simulink model "ThresholdCalibration6CH_UI"  (R2018b)
settings: Solver=VariableStepAuto  StartTime=0.0  StopTime=inf  RelTol=1e-3
libraries: simulink x16, dspstat3 x8, aerolibanimutils x1, dspnetwork x1
settings Model: Creator=Bruger  LastModifiedBy=Jonathan E. Schmidt

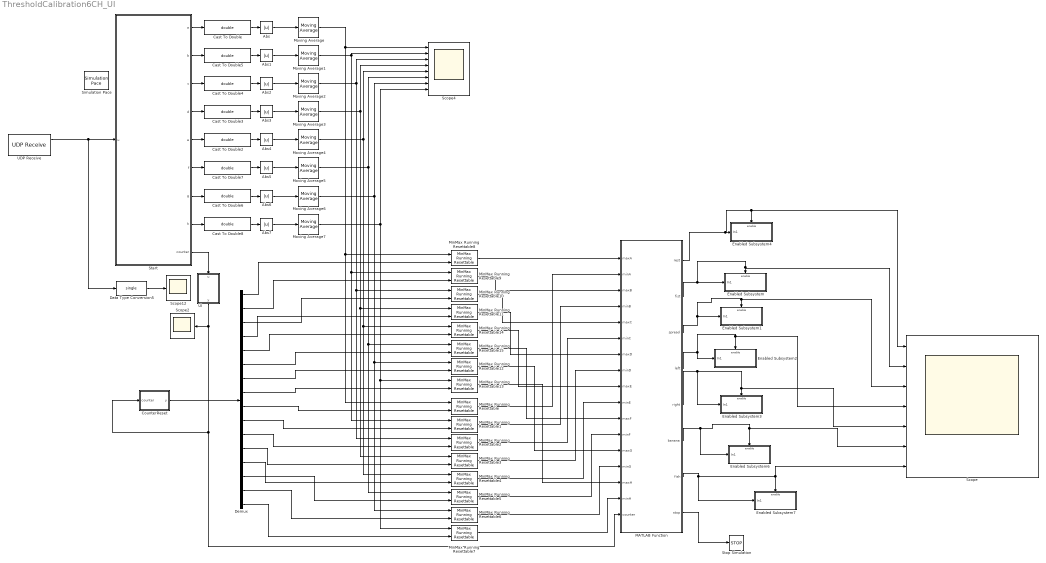
== system ThresholdCalibration6CH_UI ==
  Abs{,1..7} (8 alike) : Abs
  Cast To Double{,2..8} (8 alike) : DataTypeConversion  OutDataTypeStr=double
  "CounterReset " : MATLAB Function  TreatAsAtomicUnit=on
  Data Type Conversion5 : DataTypeConversion  OutDataTypeStr=single
  Demux : Demux  Outputs=16
  Enabled Subsystem : Subsystem  TreatAsAtomicUnit=on
  Enabled Subsystem1 : Subsystem  TreatAsAtomicUnit=on
  Enabled Subsystem2 : Subsystem  TreatAsAtomicUnit=on
  Enabled Subsystem3 : Subsystem  TreatAsAtomicUnit=on
  Enabled Subsystem4 : Subsystem  TreatAsAtomicUnit=on
  Enabled Subsystem6 : Subsystem  TreatAsAtomicUnit=on
  Enabled Subsystem7 : Subsystem  TreatAsAtomicUnit=on
  MATLAB Function : MATLAB Function  TreatAsAtomicUnit=on
  MinMax Running Resettable{,1..7} (8 alike) : simulink/Math Operations/MinMax Running Resettable  Function=min  vinit=1000
  MinMax Running Resettable{8..15} (8 alike) : simulink/Math Operations/MinMax Running Resettable  Function=max  vinit=0
  Moving Average{,1..7} (8 alike) : dspstat3/Moving Average  Method=Sliding window  ForgettingFactorPort=off  SpecifyWindowLength=on  WindowLength=50  ForgettingFactor=0.9  SimulateUsing=Code generation
  Scope : Scope  NumInputPorts=7
  Scope12 : Scope
  Scope2 : Scope
  Scope4 : Scope  NumInputPorts=8
  Simulation Pace : aerolibanimutils/Simulation Pace  SimulationPace=1  SleepMode=Auto  OutputPaceError=off  SampleTime=1/30
  "Start " : MATLAB Function  TreatAsAtomicUnit=on
  Stop Simulation : Stop
  UDP Receive : dspnetwork/UDP Receive  localURL='0.0.0.0'  localPort=54000  remoteURL='0.0.0.0'  remotePort=-1  recvBufferSize=128  dims=255  signalDatatype=int8  isVarSize=off  showBlockingTime=off  blockingTime=0  sampletime=0.02  blockPlatform=[]
      settings: SourceProductName=DSP System Toolbox  SourceProductBaseCode=DS
  UI : MATLAB Function  TreatAsAtomicUnit=on
  wires:
  UDP Receive/1 -> Data Type Conversion5/1, "Start "/1(u)
  Data Type Conversion5/1 -> Scope12/1
  Cast To Double/1 -> Abs/1
  "Start "/1(a) -> Cast To Double/1
  "Start "/2(b) -> Cast To Double5/1
  Cast To Double5/1 -> Abs1/1
  "Start "/3(c) -> Cast To Double4/1
  Cast To Double4/1 -> Abs2/1
  "Start "/4(d) -> Cast To Double3/1
  Cast To Double3/1 -> Abs3/1
  "Start "/5(e) -> Cast To Double2/1
  Cast To Double2/1 -> Abs4/1
  "Start "/6(f) -> Cast To Double7/1
  Cast To Double7/1 -> Abs5/1
  "Start "/7(g) -> Cast To Double6/1
  Cast To Double6/1 -> Abs6/1
  "Start "/8(h) -> Cast To Double8/1
  Cast To Double8/1 -> Abs7/1
  Moving Average1/1 -> MinMax Running Resettable9/1, MinMax Running Resettable1/1, Scope4/2
  Moving Average2/1 -> MinMax Running Resettable10/1, MinMax Running Resettable2/1, Scope4/3
  Moving Average3/1 -> MinMax Running Resettable11/1, MinMax Running Resettable3/1, Scope4/4
  Moving Average4/1 -> MinMax Running Resettable14/1, MinMax Running Resettable4/1, Scope4/5
  Moving Average5/1 -> MinMax Running Resettable15/1, MinMax Running Resettable5/1, Scope4/6
  Moving Average6/1 -> MinMax Running Resettable12/1, MinMax Running Resettable6/1, Scope4/7
  Moving Average7/1 -> MinMax Running Resettable7/1, MinMax Running Resettable13/1, Scope4/8
  Abs/1 -> Moving Average/1
  Abs1/1 -> Moving Average1/1
  Abs2/1 -> Moving Average2/1
  Abs3/1 -> Moving Average3/1
  Abs4/1 -> Moving Average4/1
  Abs5/1 -> Moving Average5/1
  Abs6/1 -> Moving Average6/1
  Abs7/1 -> Moving Average7/1
  MinMax Running Resettable8/1 -> MATLAB Function/1(maxA)
  MinMax Running Resettable/1 -> MATLAB Function/2(minA)
  MinMax Running Resettable9/1 -> MATLAB Function/3(maxB)
  MinMax Running Resettable1/1 -> MATLAB Function/4(minB)
  MinMax Running Resettable10/1 -> MATLAB Function/5(maxC)
  MinMax Running Resettable2/1 -> MATLAB Function/6(minC)
  MinMax Running Resettable11/1 -> MATLAB Function/7(maxD)
  MinMax Running Resettable3/1 -> MATLAB Function/8(minD)
  MinMax Running Resettable14/1 -> MATLAB Function/9(maxE)
  MinMax Running Resettable4/1 -> MATLAB Function/10(minE)
  MinMax Running Resettable15/1 -> MATLAB Function/11(maxF)
  MinMax Running Resettable5/1 -> MATLAB Function/12(minF)
  MinMax Running Resettable12/1 -> MATLAB Function/13(maxG)
  MinMax Running Resettable6/1 -> MATLAB Function/14(minG)
  MinMax Running Resettable13/1 -> MATLAB Function/15(maxH)
  MinMax Running Resettable7/1 -> MATLAB Function/16(minH)
  Demux/1 -> MinMax Running Resettable8/2
  Demux/2 -> MinMax Running Resettable9/2
  Demux/3 -> MinMax Running Resettable10/2
  Demux/4 -> MinMax Running Resettable11/2
  Demux/5 -> MinMax Running Resettable14/2
  Demux/6 -> MinMax Running Resettable15/2
  Demux/7 -> MinMax Running Resettable12/2
  Demux/8 -> MinMax Running Resettable13/2
  Demux/9 -> MinMax Running Resettable/2
  Demux/10 -> MinMax Running Resettable1/2
  Demux/11 -> MinMax Running Resettable2/2
  Demux/12 -> MinMax Running Resettable3/2
  Demux/13 -> MinMax Running Resettable4/2
  Demux/14 -> MinMax Running Resettable5/2
  Demux/15 -> MinMax Running Resettable6/2
  Demux/16 -> MinMax Running Resettable7/2
  Moving Average/1 -> MinMax Running Resettable/1, MinMax Running Resettable8/1, Scope4/1
  "CounterReset "/1(y) -> Demux/1
  MATLAB Function/2(fist) -> Scope/2, Enabled Subsystem/Enable, Enabled Subsystem/1(In1)
  MATLAB Function/3(spread) -> Scope/3, Enabled Subsystem1/Enable, Enabled Subsystem1/1(In1)
  MATLAB Function/4(left) -> Scope/4, Enabled Subsystem2/Enable, Enabled Subsystem2/1(In1)
  MATLAB Function/5(right) -> Enabled Subsystem3/1(In1), Scope/5, Enabled Subsystem3/Enable
  MATLAB Function/6(banana) -> Scope/6, Enabled Subsystem6/Enable, Enabled Subsystem6/1(In1)
  MATLAB Function/7(fish) -> Scope/7, Enabled Subsystem7/Enable, Enabled Subsystem7/1(In1)
  MATLAB Function/8(stop) -> Stop Simulation/1
  MATLAB Function/1(rest) -> Scope/1, Enabled Subsystem4/Enable, Enabled Subsystem4/1(In1)
  "Start "/9(counter) -> UI/1(u)
  UI/1(y) -> "CounterReset "/1(counter), MATLAB Function/17(counter), Scope2/1

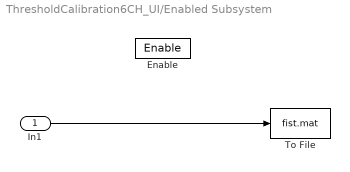
== system ThresholdCalibration6CH_UI/Enabled Subsystem ==
  In1 : Inport
  Enable : EnablePort
  To File : ToFile  Filename=fist.mat  MatrixName=fist
  wires:
  In1/1 -> To File/1

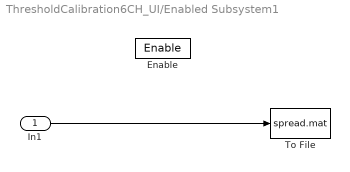
== system ThresholdCalibration6CH_UI/Enabled Subsystem1 ==
  In1 : Inport
  Enable : EnablePort
  To File : ToFile  Filename=spread.mat  MatrixName=spread
  wires:
  In1/1 -> To File/1

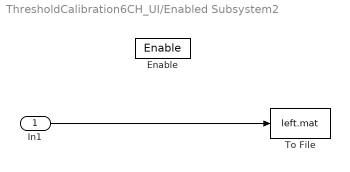
== system ThresholdCalibration6CH_UI/Enabled Subsystem2 ==
  In1 : Inport
  Enable : EnablePort
  To File : ToFile  Filename=left.mat  MatrixName=left
  wires:
  In1/1 -> To File/1

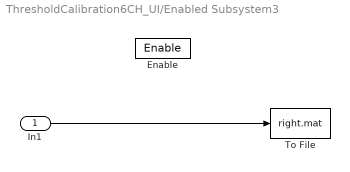
== system ThresholdCalibration6CH_UI/Enabled Subsystem3 ==
  In1 : Inport
  Enable : EnablePort
  To File : ToFile  Filename=right.mat  MatrixName=minMax
  wires:
  In1/1 -> To File/1

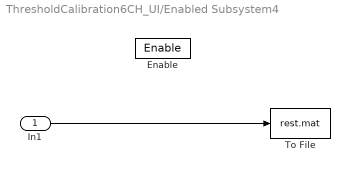
== system ThresholdCalibration6CH_UI/Enabled Subsystem4 ==
  In1 : Inport
  Enable : EnablePort
  To File : ToFile  Filename=rest.mat  MatrixName=fist
  wires:
  In1/1 -> To File/1

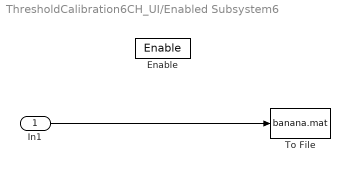
== system ThresholdCalibration6CH_UI/Enabled Subsystem6 ==
  In1 : Inport
  Enable : EnablePort
  To File : ToFile  Filename=banana.mat  MatrixName=fish
  wires:
  In1/1 -> To File/1

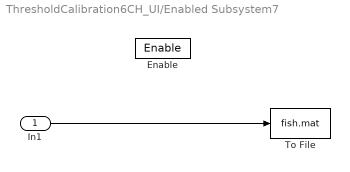
== system ThresholdCalibration6CH_UI/Enabled Subsystem7 ==
  In1 : Inport
  Enable : EnablePort
  To File : ToFile  Filename=fish.mat  MatrixName=fish
  wires:
  In1/1 -> To File/1

== matlab function ThresholdCalibration6CH_UI/UI ==
  data: u input; y output
function y = fcn(u)
coder.extrinsic('uipanel')
coder.extrinsic('uicontrol')

% persistent h1 h2 h4 counter;

persistent h1 h2 h4;


% if isempty(counter)
%     counter=0;
% else
%     counter=counter+1;
% end

if isempty(h1)
    close all;
    h1 = figure(...
    'PaperUnits','inches',...
    'Units','characters',...
    'Position',[100 20 130.4 26.8461538461538],...
    'PaperSize',[8.5 11],...
    'PaperType','usletter');

    h2 = uipanel(...
    'Parent',h1,...
    'Units','characters',...
    'Title','Current task',...
    'Position',[9.8 17.6153846153846 41.4 5.30769230769231],...
    'FontSize',10);

    h4 = uipanel(...
    'Parent',h1,...
    'Units','characters',...
    'Title','Upcoming task',...
    'Position',[9.8 9.92307692307692 41.4 5.30769230769231],...
    'FontSize',10);

    h6 = uipanel(...
    'Parent',h1,...
    'Units','characters',...
    'Title','Instructions',...
    'Position',[55.2 2.23076923076923 67.6 20.6923076923077],...
    'FontSize',10);

    h7 = uicontrol(...
    'Parent',h6,...
    'Units','characters',...
    'HorizontalAlignment','left',...
    'String',{  'The calibration process has 6 steps. Each step takes 5 seconds that are followed by 4 seconds of a rest time. The calibration starts with 10 seconds of rest. The user is expected to already be resting his/her arm once the program starts.'; blanks(0); 'The user is expected to perform the gestures in the following order:'; '1. Relaxed'; '2. Spread'; '3. Wave left'; '4. Wave right'; '5. Fist pull-back '; '6. Fist ' },...
    'Style','text',...
    'Position',[4.4 1.38461538461538 55 17.5384615384615],...
    'FontSize',9);
end

% % % % % % % % % % % % % % % % % % % % % % % % % % % % % % % % % % % % % % % % % % % % % % % % % %
% % % % % % % % % % % % % % % % % % % % % % % % % % % % % % % % % % % % % % % % % % % % % % % % % % 
% % % % % % % % % % % % % % % % % % % % % % % % % % % % % % % % % % % % % % % % % % % % % % % % % % 
% % % % % % % % % % % % % % % % % % % % % % % % % % % % % % % % % % % % % % % % % % % % % % % % % % 

switch u
    case 1
        h3 = uicontrol(...
        'Parent',h2,...
        'Units','characters',...
        'String',{  'Relaxed' },...
        'Style','text',...
        'FontSize',10,...
        'Position',[3 1.30769230769231 35 2]);
    
        h5 = uicontrol(...
        'Parent',h4,...
        'Units','characters',...
        'String',{  'Rest' },...
        'Style','text',...
        'FontSize',10,...
        'Position',[2.2 1.38461538461538 35 2]);
    
    case 250
        h3 = uicontrol(...
        'Parent',h2,...
        'Units','characters',...
        'String',{  'Rest' },...
        'Style','text',...
        'FontSize',10,...
        'Position',[3 1.30769230769231 35 2]);
    
        h5 = uicontrol(...
        'Parent',h4,...
        'Units','characters',...
        'String',{  'Spread' },...
        'Style','text',...
        'FontSize',10,...
        'Position',[2.2 1.38461538461538 35 2]);
    
    case 450
        h3 = uicontrol(...
        'Parent',h2,...
        'Units','characters',...
        'String',{  'Spread' },...
        'Style','text',...
        'FontSize',10,...
        'Position',[3 1.30769230769231 35 2]);
    
        h5 = uicontrol(...
        'Parent',h4,...
        'Units','characters',...
        'String',{  'Rest' },...
        'Style','text',...
        'FontSize',10,...
        'Position',[2.2 1.38461538461538 35 2]);
    
    case 750 
        h3 = uicontrol(...
        'Parent',h2,...
        'Units','characters',...
        'String',{  'Rest' },...
        'Style','text',...
        'FontSize',10,...
        'Position',[3 1.30769230769231 35 2]);
    
        h5 = uicontrol(...
        'Parent',h4,...
        'Units','characters',...
        'String',{  'Wave left' },...
        'Style','text',...
        'FontSize',10,...
        'Position',[2.2 1.38461538461538 35 2]);

    case 950
        h3 = uicontrol(...
        'Parent',h2,...
        'Units','characters',...
        'String',{  'Wave left' },...
        'Style','text',...
        'FontSize',10,...
        'Position',[3 1.30769230769231 35 2]);
    
        h5 = uicontrol(...
        'Parent',h4,...
        'Units','characters',...
        'String',{  'Rest' },...
        'Style','text',...
        'FontSize',10,...
        'Position',[2.2 1.38461538461538 35 2]);

    case 1250
        h3 = uicontrol(...
        'Parent',h2,...
        'Units','characters',...
        'String',{  'Rest' },...
        'Style','text',...
        'FontSize',10,...
        'Position',[3 1.30769230769231 35 2]);
    
        h5 = uicontrol(...
        'Parent',h4,...
        'Units','characters',...
        'String',{  'Wave right' },...
        'Style','text',...
        'FontSize',10,...
        'Position',[2.2 1.38461538461538 35 2]);
    
    case 1450
        h3 = uicontrol(...
        'Parent',h2,...
        'Units','characters',...
        'String',{  'Wave right' },...
        'Style','text',...
        'FontSize',10,...
        'Position',[3 1.30769230769231 35 2]);
    
        h5 = uicontrol(...
        'Parent',h4,...
        'Units','characters',...
        'String',{  'Rest' },...
        'Style','text',...
        'FontSize',10,...
        'Position',[2.2 1.38461538461538 35 2]);
    
    case 1750
        h3 = uicontrol(...
        'Parent',h2,...
        'Units','characters',...
        'String',{  'Rest' },...
        'Style','text',...
        'FontSize',10,...
        'Position',[3 1.30769230769231 35 2]);
    
        h5 = uicontrol(...
        'Parent',h4,...
        'Units','characters',...
        'String',{  'Fist pull-back' },...
        'Style','text',...
        'FontSize',10,...
        'Position',[2.2 1.38461538461538 35 2]);
    
    case 1950
        h3 = uicontrol(...
        'Parent',h2,...
        'Units','characters',...
        'String',{  'Fist pull-back' },...
        'Style','text',...
        'FontSize',10,...
        'Position',[3 1.30769230769231 35 2]);
    
        h5 = uicontrol(...
        'Parent',h4,...
        'Units','characters',...
        'String',{  'Rest' },...
        'Style','text',...
        'FontSize',10,...
        'Position',[2.2 1.38461538461538 35 2]);
    
    case 2250
        h3 = uicontrol(...
        'Parent',h2,...
        'Units','characters',...
        'String',{  'Rest' },...
        'Style','text',...
        'FontSize',10,...
        'Position',[3 1.30769230769231 35 2]);
    
        h5 = uicontrol(...
        'Parent',h4,...
        'Units','characters',...
        'String',{  'Fist' },...
        'Style','text',...
        'FontSize',10,...
        'Position',[2.2 1.38461538461538 35 2]);
    
    case 2450
        h3 = uicontrol(...
        'Parent',h2,...
        'Units','characters',...
        'String',{  'Fist' },...
        'Style','text',...
        'FontSize',10,...
        'Position',[3 1.30769230769231 35 2]);
    
        h5 = uicontrol(...
        'Parent',h4,...
        'Units','characters',...
        'String',{  '-' },...
        'Style','text',...
        'FontSize',10,...
        'Position',[2.2 1.38461538461538 35 2]);
    
    case 2750
        h3 = uicontrol(...
        'Parent',h2,...
        'Units','characters',...
        'String',{  'Calibration is done!' },...
        'Style','text',...
        'FontSize',10,...
        'Position',[3 1.30769230769231 35 2]);
    
        h5 = uicontrol(...
        'Parent',h4,...
        'Units','characters',...
        'String',{  'Calibration is done!' },...
        'Style','text',...
        'FontSize',10,...
        'Position',[2.2 1.38461538461538 35 2]);
end
        
y = u;

== matlab function ThresholdCalibration6CH_UI/Start  ==
  data: u input; a output; b output; c output; d output; e output; f output; g output; h output; counter output
%a is the output of this block, and fcn(u) is the input required
function [a,b,c,d,e,f,g,h,counter]  = fcn(u)

persistent count 
if isempty(count)
   count =0; 
end

% We could error message in case we are receiving zero vector
if isempty(u)==0  
   count = count+1; 
end

counter=count;
%Below the output a is specified as the 3 row of the 8x1 input vector u
a = u(1,:);
b = u(2,:);
c = u(3,:);
d = u(4,:);
e = u(5,:);
f = u(6,:);
g = u(7,:);
h = u(8,:);

% a = u(1);
% b = u(2);
% c = u(3);
% d = u(4);
% e = u(5);
% f = u(6);
% g = u(7);
% h = u(8);

== matlab function ThresholdCalibration6CH_UI/MATLAB Function ==
  data: rest output; maxA input; minA input; maxB input; minB input; maxC input; minC input; maxD input; minD input; maxE input; minE input; maxF input; minF input; maxG input; minG input; maxH input; minH input; fist output; counter input; spread output; left output; right output; banana output; fish output; stop output
function [rest,fist,spread,left,right,banana,fish, stop] = fcn(maxA, minA, maxB, minB, maxC, minC, maxD, minD, maxE, minE, maxF, minF, maxG, minG, maxH, minH, counter)
    
    stop=0;
    rest=zeros(1,16);
    fist=zeros(1,16);
    spread=zeros(1,16);
    left=zeros(1,16);
    right=zeros(1,16);
    banana=zeros(1,16);
    fish=zeros(1,16);

if counter==250
    rest=[maxA minA maxB minB maxC minC maxD minD maxE minE maxF minF maxG minG maxH minH];

elseif counter==750
    fist=[maxA minA maxB minB maxC minC maxD minD maxE minE maxF minF maxG minG maxH minH];

elseif counter==1250
    spread=[maxA minA maxB minB maxC minC maxD minD maxE minE maxF minF maxG minG maxH minH];

elseif counter==1750
    left=[maxA minA maxB minB maxC minC maxD minD maxE minE maxF minF maxG minG maxH minH];
    
elseif counter==2250
    right=[maxA minA maxB minB maxC minC maxD minD maxE minE maxF minF maxG minG maxH minH];
    
elseif counter==2750
    banana=[maxA minA maxB minB maxC minC maxD minD maxE minE maxF minF maxG minG maxH minH];
    
elseif counter==3250
    fish=[maxA minA maxB minB maxC minC maxD minD maxE minE maxF minF maxG minG maxH minH];    
    pause(0.5);
    stop=1;
     
end

== matlab function ThresholdCalibration6CH_UI/CounterReset  ==
  data: counter input; y output
function y = fcn(counter)
if counter==50
    y=[1 1 1 1 1 1 1 1 1 1 1 1 1 1 1 1];
elseif counter==550
    y=[1 1 1 1 1 1 1 1 1 1 1 1 1 1 1 1];
elseif counter==1050
    y=[1 1 1 1 1 1 1 1 1 1 1 1 1 1 1 1];
elseif counter==1550
    y=[1 1 1 1 1 1 1 1 1 1 1 1 1 1 1 1];
elseif counter==2050
    y=[1 1 1 1 1 1 1 1 1 1 1 1 1 1 1 1];
elseif counter==2550
    y=[1 1 1 1 1 1 1 1 1 1 1 1 1 1 1 1];

    
else 
    y=zeros(1,16)
end
